simulink library "lbr4p_joint_impctrl_test_lib"  (Simulink 9.0)
settings: Solver=VariableStepAuto  StartTime=0.0  StopTime=10.0  RelTol=1e-3
undefined symbols (not defined in the file): T1_filter_input
settings Model: SuppressorTable=22 serialization::archive 11 0 6 0 0 0 11 0  Creator=schappler  LastModifiedBy=schappler

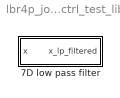
== system lbr4p_joint_impctrl_test_lib ==
  7D low pass filter : Subsystem  mask{f=T1_filter_input}
      mask prompts: f "T1"

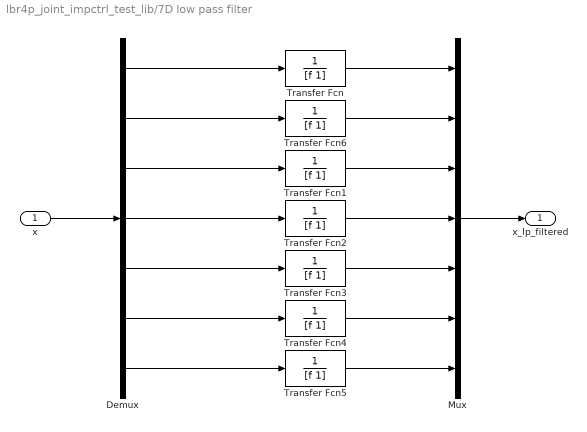
== system lbr4p_joint_impctrl_test_lib/7D low pass filter ==
  x : Inport  PortDimensions=7
  Demux : Demux  Outputs=7
  Mux : Mux  Inputs=7
  Transfer Fcn{,1..6} (7 alike) : TransferFcn  Denominator=[f 1]
  x_lp_filtered : Outport  PortDimensions=7
  wires:
  Transfer Fcn6/1 -> Mux/2
  Demux/2 -> Transfer Fcn6/1
  Transfer Fcn/1 -> Mux/1
  Demux/1 -> Transfer Fcn/1
  Mux/1 -> x_lp_filtered/1
  x/1 -> Demux/1
  Transfer Fcn1/1 -> Mux/3
  Demux/3 -> Transfer Fcn1/1
  Demux/4 -> Transfer Fcn2/1
  Transfer Fcn2/1 -> Mux/4
  Demux/5 -> Transfer Fcn3/1
  Transfer Fcn3/1 -> Mux/5
  Demux/6 -> Transfer Fcn4/1
  Transfer Fcn4/1 -> Mux/6
  Demux/7 -> Transfer Fcn5/1
  Transfer Fcn5/1 -> Mux/7
